simulink model "K_discrete_continuous_comp"  (R2022b)
settings: Solver=VariableStepAuto  StartTime=0.0  StopTime=2  RelTol=1e-3
settings Model: Creator=isaac  LastModifiedBy=isaac
settings DebuggingCC: AlgebraicLoopMsg=error  UnconnectedInputMsg=warning  UnconnectedOutputMsg=warning  UnconnectedLineMsg=warning
settings ModelReferenceCC: EnableRefExpFcnMdlSchedulingChecks=on
settings RTWCC: DLArmComputeVersion=19.05

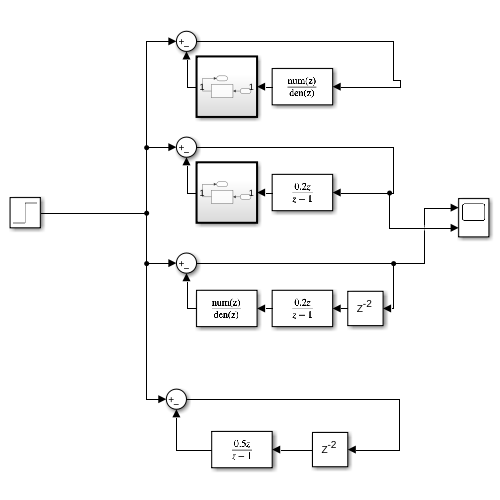
[thumbnail: Simulink's stored preview of the top-level diagram]
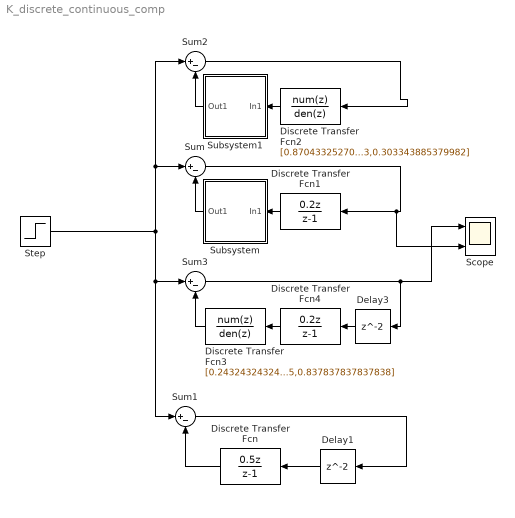
== system K_discrete_continuous_comp ==
  Delay1 : Delay  SampleTime=0.01
  Delay3 : Delay  SampleTime=0.001
  Discrete Transfer Fcn : DiscreteTransferFcn  Numerator=[0.5 0]  Denominator=[1 -1]  SampleTime=0.01
  Discrete Transfer Fcn1 : DiscreteTransferFcn  Numerator=[0.2 0]  Denominator=[1 -1]  SampleTime=0.001
  Discrete Transfer Fcn2 : DiscreteTransferFcn  Numerator=[0.870433252701781,-1.41605292874724,1.81539473367975,-1.37279099039499,0.669476422405778,-0.244920931458109]  Denominator=[1,-1.47847153282669,0.549088840442877,-0.184065302942944,-0.189895890053223,0.303343885379982]  SampleTime=0.001
  Discrete Transfer Fcn3 : DiscreteTransferFcn  Numerator=[0.243243243243243,0.486486486486487,0.243243243243243]  Denominator=[1,-0.864864864864865,0.837837837837838]  SampleTime=0.001
  Discrete Transfer Fcn4 : DiscreteTransferFcn  Numerator=[0.2 0]  Denominator=[1 -1]  SampleTime=0.001
  Scope : Scope  NumInputPorts=2
  Step : Step  Before=1  SampleTime=0
  Subsystem : Subsystem  TreatAsAtomicUnit=on
  Subsystem1 : Subsystem  TreatAsAtomicUnit=on
  Sum{,1..3} (4 alike) : Sum  Inputs=|+-
  wires:
  Sum1/1 -> Delay1/1
  Discrete Transfer Fcn/1 -> Sum1/2
  Sum/1 -> Scope/2, Discrete Transfer Fcn1/1
  Discrete Transfer Fcn1/1 -> Subsystem/1(In1)
  Subsystem/1(Out1) -> Sum/2
  Delay1/1 -> Discrete Transfer Fcn/1
  Subsystem1/1(Out1) -> Sum2/2
  Discrete Transfer Fcn2/1 -> Subsystem1/1(In1)
  Sum3/1 -> Scope/1, Delay3/1
  Delay3/1 -> Discrete Transfer Fcn4/1
  Discrete Transfer Fcn3/1 -> Sum3/2
  Discrete Transfer Fcn4/1 -> Discrete Transfer Fcn3/1
  Step/1 -> Sum3/1, Sum1/1, Sum2/1, Sum/1
  Sum2/1 -> Discrete Transfer Fcn2/1

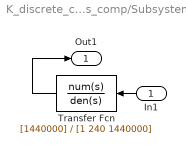
== system K_discrete_continuous_comp/Subsystem ==
  In1 : Inport
  Transfer Fcn : TransferFcn  Numerator=[1440000]  Denominator=[1 240 1440000]
  Out1 : Outport
  wires:
  Transfer Fcn/1 -> Out1/1
  In1/1 -> Transfer Fcn/1

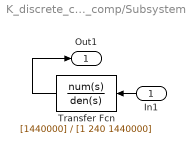
== system K_discrete_continuous_comp/Subsystem1 ==
  In1 : Inport
  Transfer Fcn : TransferFcn  Numerator=[1440000]  Denominator=[1 240 1440000]
  Out1 : Outport
  wires:
  Transfer Fcn/1 -> Out1/1
  In1/1 -> Transfer Fcn/1
